simulink model "gyak10_matlabgyak2_sim_UJRAOLDVA"  (R2016a)
settings: Solver=ode45  StartTime=0.0  StopTime=40  MaxStep=0.01  RelTol=1e-3
settings Model: Creator=ppolcz  LastModifiedBy=ppolcz
settings DataIOCC: LimitDataPoints=on  SaveFormat=Array
settings HardwareCC: ProdBitPerPointer=32  ProdLargestAtomicFloat=None  ProdIntDivRoundTo=Undefined  ProdEndianess=Unspecified  ProdWordSize=32  ProdHWDeviceType=32-bit Generic
settings ModelReferenceCC: PropagateSignalLabelsOutOfModel=off
settings ConfigComp: CovModelRefEnable=Off

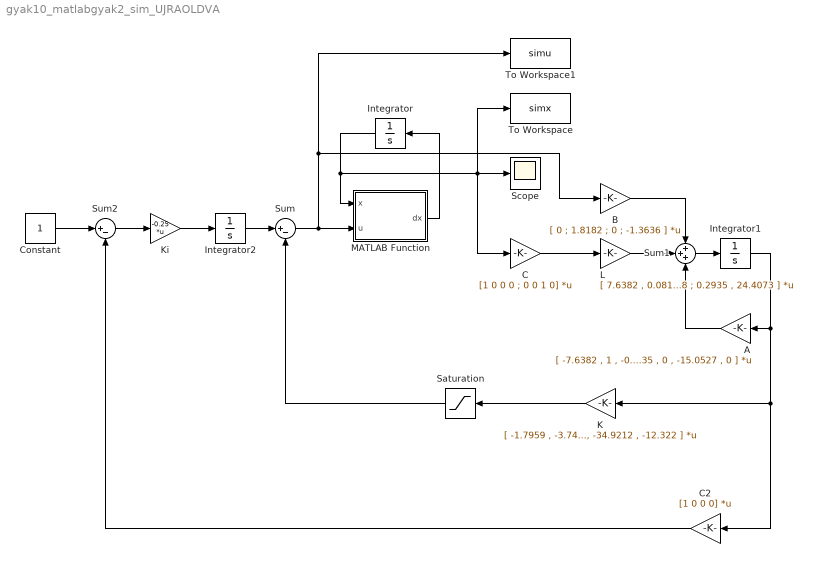
== system gyak10_matlabgyak2_sim_UJRAOLDVA ==
  A : Gain  Gain=[ -7.6382 , 1 , -0.0811 , 0 ; -14.5773 , -0 , -0.3123 , 0 ; -0.0761 , 0 , -7.7618 , 1 ; -0.2935 , 0 , -15.0527 , 0 ]  Multiplication=Matrix(K*u)
  B : Gain  Gain=[ 0 ; 1.8182 ; 0 ; -1.3636 ]  Multiplication=Matrix(K*u)
  C : Gain  Gain=[1 0 0 0 ; 0 0 1 0]  Multiplication=Matrix(K*u)
  C2 : Gain  Gain=[1 0 0 0]  Multiplication=Matrix(K*u)
  Constant : Constant
  Integrator : Integrator  InitialCondition=[0,0,0.3,0]'
  Integrator1 : Integrator  InitialCondition=[0,0,0.4,0]'
  Integrator2 : Integrator
  K : Gain  Gain=[ -1.7959 , -3.7415 , -34.9212 , -12.322 ]  Multiplication=Matrix(K*u)
  Ki : Gain  Gain=-0.25  Multiplication=Matrix(K*u)
  L : Gain  Gain=[ 7.6382 , 0.0811 ; 14.5773 , -2.3605 ; 0.0761 , 7.7618 ; 0.2935 , 24.4073 ]  Multiplication=Matrix(K*u)
  MATLAB Function : MATLAB Function  TreatAsAtomicUnit=on
  Saturation : Saturate  UpperLimit=10  LowerLimit=-10
  Scope : Scope
  Sum : Sum  Inputs=|+-
  Sum1 : Sum  Inputs=+++
  Sum2 : Sum  Inputs=|+-
  To Workspace : ToWorkspace  VariableName=simx  SaveFormat=Timeseries  SampleTime=-1
  To Workspace1 : ToWorkspace  VariableName=simu  SaveFormat=Timeseries  SampleTime=-1
  wires:
  MATLAB Function/1(dx) -> Integrator/1
  Integrator/1 -> C/1, To Workspace/1, Scope/1, MATLAB Function/1(x)
  Sum/1 -> B/1, To Workspace1/1, MATLAB Function/2(u)
  C/1 -> L/1
  B/1 -> Sum1/1
  L/1 -> Sum1/2
  A/1 -> Sum1/3
  Sum1/1 -> Integrator1/1
  Integrator1/1 -> C2/1, K/1, A/1
  K/1 -> Saturation/1
  Saturation/1 -> Sum/2
  C2/1 -> Sum2/2
  Integrator2/1 -> Sum/1
  Sum2/1 -> Ki/1
  Ki/1 -> Integrator2/1
  Constant/1 -> Sum2/1

== matlab function gyak10_matlabgyak2_sim_UJRAOLDVA/MATLAB Function ==
  data: x input; u input; dx output
function dx = fcn(x,u)
%#codegen

% model parameters
M = 0.5;
m = 0.2;
l = 1;
g = 9.8;
b = 0;

v = x(2);
phi = x(3);
omega = x(4);

q = 4*(M+m) - 3*m*cos(phi)^2;

f = [
    v
    (4*m*l*sin(phi)*omega^2 - 1.5*m*g*sin(2*phi) -4*b*v) / q
    omega
    3*(-m*l*sin(2*phi)*omega^2 / 2 + (M+m)*g*sin(phi) + b*cos(phi)*v) / (l*q)
    ];

g = [
    0
    4*l
    0
    -3*cos(phi)
    ] / (l*q);

dx = f + g*u;
